simulink model "stepRecovery"  (Simulink 8.8)
settings: Solver=FixedStepDiscrete  StartTime=0.0  StopTime="CONFIG.SIMULATION_TIME "  FixedStep=CONFIG.Ts  RelTol=1e-3
InitFcn:
  | cd(fileparts(which(bdroot)));
  | initStepRecovery;
undefined symbols (not defined in the file or in its folder): bVectorConstraints, bVectorConstraintsMPC, CONFIG, ConstraintsMatrix, ConstraintsMatrixMPC, DiscIntNeverNeededParam, gain, mpc_init, reg, ROBOT_DOF, ROBOT_DOF_FOR_SIMULINK, sat, sm, WBT_robotName
libraries: WBToolboxLibrary x112, simulink x13, simulink_extras x4
(part 1 of 4)
settings Model: SuppressorTable=22 serialization::archive 11 0 3 0 0 0 11 0  Creator=daniele  LastModifiedBy=sdafarra
settings DataIOCC: SignalLoggingSaveFormat=Dataset
settings OptimizationCC: ExpressionDepthLimit=2147483647
settings DebuggingCC: SignalInfNanChecking=warning  UnderspecifiedInitializationDetection=Simplified  MergeDetectMultiDrivingBlocksExec=error  SolverPrmCheckMsg=warning  MultiTaskCondExecSysMsg=warning  SingleTaskRateTransMsg=warning  CheckMatrixSingularityMsg=warning  AllowSymbolicDim=off
settings SFSimCC: SimParseCustomCode=off

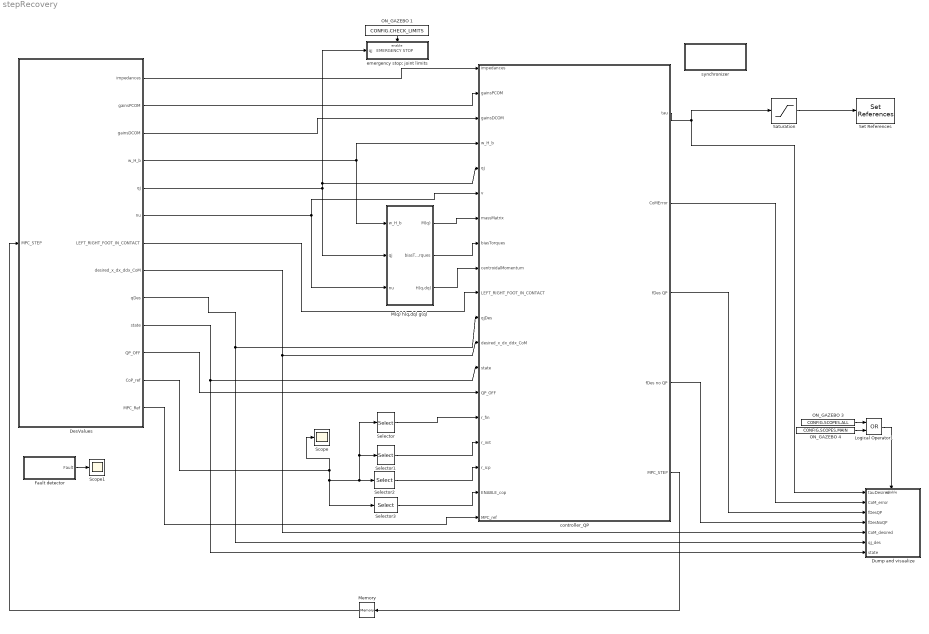
== system stepRecovery ==
  DesValues : Subsystem  Priority=-10
  Dump and visualize : Subsystem
  Fault detector : Subsystem
  Logical Operator1 : Logic  Operator=OR  AllPortsSameDT=off  OutDataTypeStr=boolean
  M(q) h(q,dq) g(q) : Subsystem
  Memory : Memory
  ON_GAZEBO 1 : Constant  Value=CONFIG.CHECK_LIMITS
  ON_GAZEBO 3 : Constant  Value=CONFIG.SCOPES.ALL
  ON_GAZEBO 4 : Constant  Value=CONFIG.SCOPES.MAIN
  Saturation : Saturate  UpperLimit=sat.torque  LowerLimit=-sat.torque
  Scope : Scope
  Scope1 : Scope
  Selector : Selector  InputPortWidth=10  IndexOptions=Index vector (dialog)  Indices=[1:3]  OutputSizes=1
  Selector1 : Selector  InputPortWidth=10  IndexOptions=Index vector (dialog)  Indices=[4:6]  OutputSizes=1
  Selector2 : Selector  InputPortWidth=10  IndexOptions=Index vector (dialog)  Indices=[7:9]  OutputSizes=1
  Selector3 : Selector  InputPortWidth=10  IndexOptions=Index vector (dialog)  Indices=[10]  OutputSizes=1
  Set References : WBToolboxLibrary/wholeBodyActuators/Set References  controlType=Torque  fullOrSubControl=Full  controlledJoints=''  robotName=WBT_robotName  localName=WBT_modelName  wbiFile=WBT_wbiFilename  wbiList=WBT_wbiList
  controller_QP : Subsystem
  emergency stop: joint limits : Subsystem
  synchronizer : Subsystem
      mask Display: disp('SYNCHRONIZER')
  wires:
  M(q) h(q,dq) g(q)/1(M(q)) -> controller_QP/7(massMatrix)
  DesValues/5(qj) -> M(q) h(q,dq) g(q)/2(qj), controller_QP/5(qj), emergency stop: joint limits/1(qj   EMERGENCY STOP)
  M(q) h(q,dq) g(q)/2(biasTorques) -> controller_QP/8(biasTorques)
  M(q) h(q,dq) g(q)/3(H(q,dq)) -> controller_QP/9(centroidalMomentum)
  controller_QP/1("tau ") -> Saturation/1, Dump and visualize/1(tauDesired)
  controller_QP/2(CoMError) -> Dump and visualize/2(CoM_error)
  DesValues/9(qDes) -> Dump and visualize/6(qj_des), controller_QP/11(qjDes)
  DesValues/7(LEFT_RIGHT_FOOT_IN_CONTACT) -> controller_QP/10(LEFT_RIGHT_FOOT_IN_CONTACT)
  DesValues/8(desired_x_dx_ddx_CoM) -> Dump and visualize/5(CoM_desired), controller_QP/12(desired_x_dx_ddx_CoM)
  DesValues/1(impedances) -> controller_QP/1(impedances)
  DesValues/4(w_H_b) -> M(q) h(q,dq) g(q)/1(w_H_b), controller_QP/4(w_H_b)
  DesValues/6(nu) -> M(q) h(q,dq) g(q)/3(nu), controller_QP/6(v)
  Logical Operator1/1 -> Dump and visualize/Enable
  DesValues/10(state) -> Dump and visualize/7(state), controller_QP/13("state ")
  controller_QP/4(fDes no QP) -> Dump and visualize/4(fDesNoQP)
  controller_QP/3(fDes QP) -> Dump and visualize/3(fDesQP)
  ON_GAZEBO 1/1 -> emergency stop: joint limits/Enable
  ON_GAZEBO 3/1 -> Logical Operator1/1
  ON_GAZEBO 4/1 -> Logical Operator1/2
  DesValues/2(gainsPCOM) -> controller_QP/2(gainsPCOM)
  DesValues/3(gainsDCOM) -> controller_QP/3(gainsDCOM)
  DesValues/11("QP_OFF ") -> controller_QP/14(QP_OFF)
  Saturation/1 -> Set References/1
  Selector2/1 -> controller_QP/17(r_icp)
  Selector1/1 -> controller_QP/16(r_init)
  Selector/1 -> controller_QP/15(r_fin)
  Selector3/1 -> controller_QP/18(ENABLE_cop)
  DesValues/12(CoP_ref) -> Selector1/1, Selector/1, Selector2/1, Selector3/1, Scope/1
  DesValues/13(MPC_Ref) -> controller_QP/19(MPC_ref)
  Fault detector/1("Fault ") -> Scope1/1
  controller_QP/5(MPC_STEP) -> Memory/1
  Memory/1 -> DesValues/1(MPC_STEP)

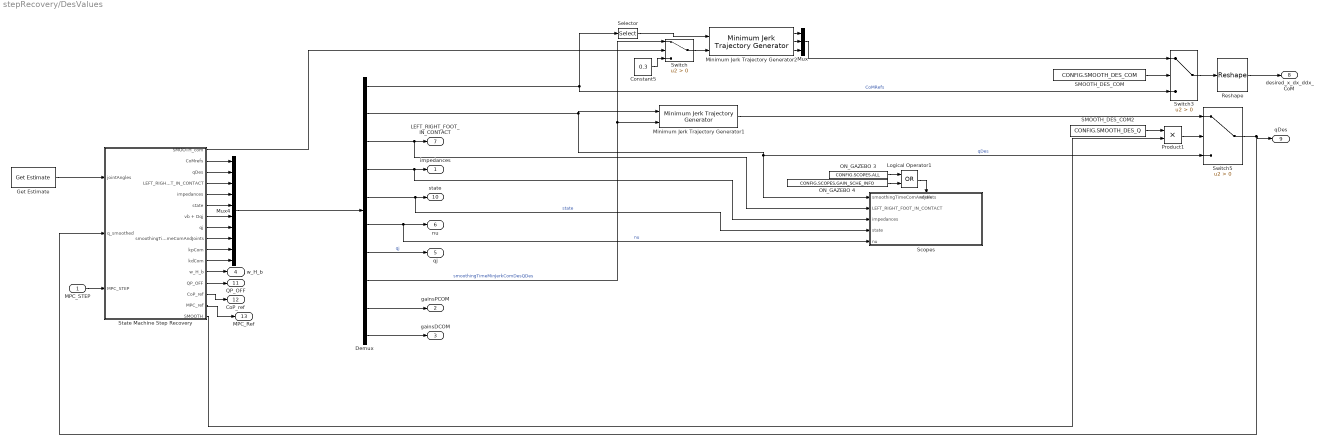
== system stepRecovery/DesValues ==
  MPC_STEP : Inport
  Constant5 : Constant  Value=0.3
  Demux : Demux  Outputs=[9,ROBOT_DOF,2,ROBOT_DOF,1,ROBOT_DOF+6,ROBOT_DOF,1,3,3]
  Get Estimate : WBToolboxLibrary/wholeBodyStates/Get Estimate  estimateType=Joints Position  robotName=WBT_robotName  localName=WBT_modelName  wbiFile=WBT_wbiFilename  wbiList=WBT_wbiList
  Logical Operator1 : Logic  Operator=OR  AllPortsSameDT=off  OutDataTypeStr=boolean
  Minimum Jerk Trajectory Generator1 : WBToolboxLibrary/Utilities/Minimum Jerk Trajectory Generator  externalSettlingTime=on  settlingTime=1  sampleTime=CONFIG.Ts  resetOnSettlingTime=off  firstDerivatives=off  secondDerivatives=off  explicitInitialValue=off
  Minimum Jerk Trajectory Generator2 : WBToolboxLibrary/Utilities/Minimum Jerk Trajectory Generator  externalSettlingTime=on  settlingTime=references.com.smoothingTime  sampleTime=CONFIG.Ts  resetOnSettlingTime=off  firstDerivatives=on  secondDerivatives=on  explicitInitialValue=off
  Mux : Mux  Inputs=3
  Mux4 : Mux  Inputs=10
  ON_GAZEBO 3 : Constant  Value=CONFIG.SCOPES.ALL
  ON_GAZEBO 4 : Constant  Value=CONFIG.SCOPES.GAIN_SCHE_INFO
  Product1 : Product
  Reshape : Reshape  OutputDimensionality=Customize  OutputDimensions=[3,3]
  SMOOTH_DES_COM : Constant  Value=CONFIG.SMOOTH_DES_COM
  SMOOTH_DES_COM2 : Constant  Value=CONFIG.SMOOTH_DES_Q
  "Scopes  " : Subsystem
  Selector : Selector  InputPortWidth=9  IndexOptions=Index vector (dialog)  Indices=[1 2 3]  OutputSizes=1
  State Machine Step Recovery : Subsystem  Priority=-100
  Switch : Switch  Criteria=u2 > Threshold
  Switch3 : Switch  Criteria=u2 > Threshold
  Switch5 : Switch  Criteria=u2 > Threshold
  impedances : Outport
  gainsPCOM : Outport  Port=2
  gainsDCOM : Outport  Port=3
  w_H_b : Outport  Port=4
  qj : Outport  Port=5
  nu : Outport  Port=6
  LEFT_RIGHT_FOOT_IN_CONTACT : Outport  Port=7
  desired_x_dx_ddx_CoM : Outport  Port=8
  qDes : Outport  Port=9
  state : Outport  Port=10
  "QP_OFF " : Outport  Port=11
  CoP_ref : Outport  Port=12
  MPC_Ref : Outport  Port=13
  wires:
  Reshape/1 -> desired_x_dx_ddx_CoM/1
  Minimum Jerk Trajectory Generator2/1 -> Mux/1
  Minimum Jerk Trajectory Generator2/2 -> Mux/2
  Minimum Jerk Trajectory Generator2/3 -> Mux/3
  Switch3/1 -> Reshape/1
  Switch5/1 -> State Machine Step Recovery/2("q_smoothed "), qDes/1
  Demux/7 -> qj/1  "qj"
  State Machine Step Recovery/12(w_H_b) -> w_H_b/1
  Demux/5 -> "Scopes  "/4(state), state/1  "state"
  Demux/8 -> Switch/1, Minimum Jerk Trajectory Generator1/2  "smoothingTimeMinJerkComDesQDes"
  Logical Operator1/1 -> "Scopes  "/Enable
  Demux/1 -> Selector/1, Switch3/3  "CoMRefs"
  Mux/1 -> Switch3/1
  Selector/1 -> Minimum Jerk Trajectory Generator2/1
  Demux/2 -> Minimum Jerk Trajectory Generator1/1, "Scopes  "/1(smoothingTimeComAndJoints), Switch5/3  "qDes"
  Minimum Jerk Trajectory Generator1/1 -> Switch5/1
  ON_GAZEBO 3/1 -> Logical Operator1/1
  ON_GAZEBO 4/1 -> Logical Operator1/2
  Demux/6 -> nu/1, "Scopes  "/5(nu)  "nu"
  Mux4/1 -> Demux/1
  Demux/4 -> "Scopes  "/3(impedances), impedances/1
  Demux/3 -> "Scopes  "/2(LEFT_RIGHT_FOOT_IN_CONTACT), LEFT_RIGHT_FOOT_IN_CONTACT/1
  Demux/9 -> gainsPCOM/1
  Demux/10 -> gainsDCOM/1
  State Machine Step Recovery/4(LEFT_RIGHT_FOOT_IN_CONTACT) -> Mux4/3
  State Machine Step Recovery/3(qDes) -> Mux4/2
  State Machine Step Recovery/2(CoMrefs) -> Mux4/1
  State Machine Step Recovery/5(impedances) -> Mux4/4
  State Machine Step Recovery/6(state) -> Mux4/5
  State Machine Step Recovery/7(vb + Dqj) -> Mux4/6
  State Machine Step Recovery/8(qj) -> Mux4/7
  State Machine Step Recovery/9(smoothingTimeComAndJoints) -> Mux4/8
  Get Estimate/1 -> State Machine Step Recovery/1(jointAngles)
  State Machine Step Recovery/10(kpCom) -> Mux4/9
  State Machine Step Recovery/11(kdCom) -> Mux4/10
  State Machine Step Recovery/13(QP_OFF) -> "QP_OFF "/1
  SMOOTH_DES_COM/1 -> Switch3/2
  SMOOTH_DES_COM2/1 -> Product1/1
  Product1/1 -> Switch5/2
  State Machine Step Recovery/16(SMOOTH) -> Product1/2
  State Machine Step Recovery/1(SMOOTH_com) -> Switch/2
  Switch/1 -> Minimum Jerk Trajectory Generator2/2
  Constant5/1 -> Switch/3
  State Machine Step Recovery/14(CoP_ref) -> CoP_ref/1
  State Machine Step Recovery/15(MPC_ref) -> MPC_Ref/1
  MPC_STEP/1 -> State Machine Step Recovery/3(MPC_STEP)

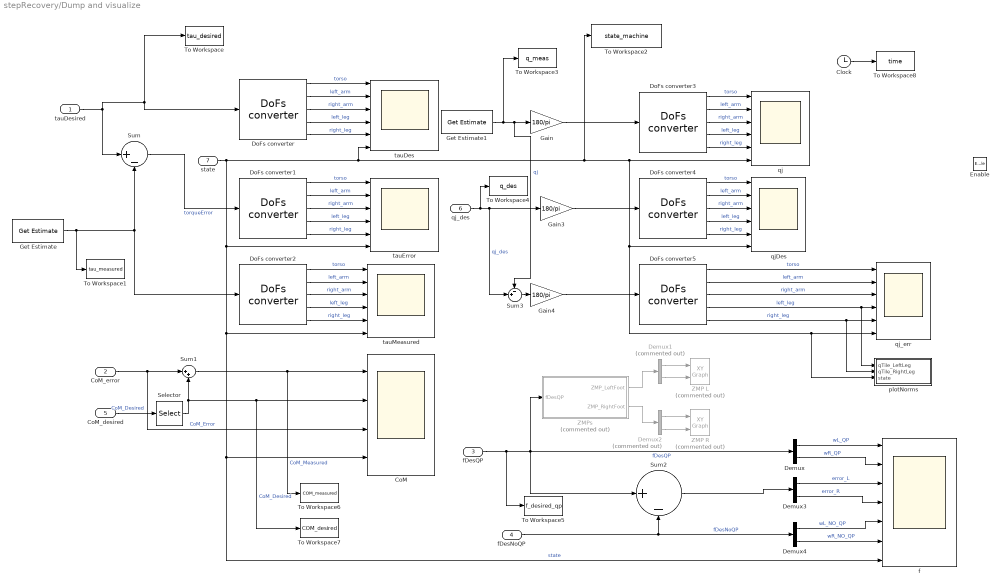
== system stepRecovery/Dump and visualize ==
  tauDesired : Inport
  CoM_error : Inport  Port=2
  fDesQP : Inport  Port=3
  fDesNoQP : Inport  Port=4
  CoM_desired : Inport  Port=5
  qj_des : Inport  Port=6
  state : Inport  Port=7
  Enable : EnablePort
  Clock : Clock
  CoM : Scope  NumInputPorts=4
  Demux : Demux  Outputs=2
  Demux1 : Demux  Commented=on  Outputs=2
  Demux2 : Demux  Commented=on  Outputs=2
  Demux3 : Demux  Outputs=2
  Demux4 : Demux  Outputs=2
  DoFs converter{,1..5} (6 alike) : WBToolboxLibrary/Utilities/DoFs converter  yarp2WBIOption=From WBI to YARP  robotName=WBT_robotName  localName=WBT_modelName  wbiFile=WBT_wbiFilename  wbiList=WBT_wbiList
  Gain : Gain  Gain=180/pi
  Gain3 : Gain  Gain=180/pi
  Gain4 : Gain  Gain=180/pi
  Get Estimate : WBToolboxLibrary/wholeBodyStates/Get Estimate  estimateType=Joints Torque  robotName=WBT_robotName  localName=WBT_modelName  wbiFile=WBT_wbiFilename  wbiList=WBT_wbiList
  Get Estimate1 : WBToolboxLibrary/wholeBodyStates/Get Estimate  estimateType=Joints Position  robotName=WBT_robotName  localName=WBT_modelName  wbiFile=WBT_wbiFilename  wbiList=WBT_wbiList
  Selector : Selector  NumberOfDimensions=2  IndexOptions=Index vector (dialog),Index vector (dialog)  Indices=[1:3],1  OutputSizes=1,1
  Sum : Sum  Inputs=|+-
  Sum1 : Sum  Inputs=|++
  Sum2 : Sum  Inputs=|+-
  Sum3 : Sum  Inputs=-+|
  To Workspace : ToWorkspace  VariableName=tau_desired  SampleTime=-1
      settings: Save2DSignal=2-D array (concatenate along first dimension)
  To Workspace1 : ToWorkspace  VariableName=tau_measured  SampleTime=-1
      settings: Save2DSignal=2-D array (concatenate along first dimension)
  To Workspace2 : ToWorkspace  VariableName=state_machine  SampleTime=-1
  To Workspace3 : ToWorkspace  VariableName=q_meas  SampleTime=-1
  To Workspace4 : ToWorkspace  VariableName=q_des  SampleTime=-1
  To Workspace5 : ToWorkspace  VariableName=f_desired_qp  SampleTime=-1
      settings: Save2DSignal=2-D array (concatenate along first dimension)
  To Workspace6 : ToWorkspace  VariableName=COM_measured  SampleTime=-1
  To Workspace7 : ToWorkspace  VariableName=COM_desired  SampleTime=-1
  To Workspace8 : ToWorkspace  VariableName=time  SampleTime=-1
  ZMP L : simulink/Sinks/XY Graph  Commented=on  xmin=gain.footSize(1,1)  xmax=gain.footSize(1,2)  ymin=gain.footSize(2,1)  ymax=gain.footSize(2,2)  st=-1
  ZMP R : simulink/Sinks/XY Graph  Commented=on  xmin=gain.footSize(1,1)  xmax=gain.footSize(1,2)  ymin=gain.footSize(2,1)  ymax=gain.footSize(2,2)  st=-1
  ZMPs : Subsystem  Commented=on
  f : Scope  NumInputPorts=7
  plotNorms : Subsystem
  qj : Scope  NumInputPorts=6
  qjDes : Scope  NumInputPorts=6
  qj_err : Scope  NumInputPorts=6
  tauDes : Scope  NumInputPorts=6
  tauError : Scope  NumInputPorts=6
  tauMeasured : Scope  NumInputPorts=6
  wires:
  CoM_error/1 -> Sum1/1, CoM/3  "CoM_Error"
  CoM_desired/1 -> Selector/1  "CoM_Desired"
  Sum1/1 -> To Workspace6/1, CoM/1  "CoM_Measured"
  Get Estimate1/1 -> To Workspace3/1, Sum3/1, Gain/1  "qj"
  Gain/1 -> DoFs converter3/1
  DoFs converter3/5 -> qj/5  "right_leg"
  DoFs converter3/1 -> qj/1  "torso"
  DoFs converter3/2 -> qj/2  "left_arm"
  DoFs converter3/4 -> qj/4  "left_leg"
  DoFs converter3/3 -> qj/3  "right_arm"
  fDesQP/1 -> To Workspace5/1, Demux/1, ZMPs/1(fDesQP), Sum2/1  "fDesQP"
  ZMPs/1(ZMP_LeftFoot) -> Demux1/1
  ZMPs/2(ZMP_RightFoot) -> Demux2/1
  Demux1/1 -> ZMP L/1
  Demux1/2 -> ZMP L/2
  Demux2/1 -> ZMP R/1
  Demux2/2 -> ZMP R/2
  Sum2/1 -> Demux3/1
  fDesNoQP/1 -> Demux4/1, Sum2/2  "fDesNoQP"
  tauDesired/1 -> DoFs converter/1, To Workspace/1, Sum/1
  Get Estimate/1 -> To Workspace1/1, DoFs converter2/1, Sum/2
  DoFs converter/5 -> tauDes/5  "right_leg"
  DoFs converter/1 -> tauDes/1  "torso"
  DoFs converter/2 -> tauDes/2  "left_arm"
  DoFs converter/4 -> tauDes/4  "left_leg"
  DoFs converter/3 -> tauDes/3  "right_arm"
  DoFs converter1/5 -> tauError/5  "right_leg"
  DoFs converter1/1 -> tauError/1  "torso"
  DoFs converter1/2 -> tauError/2  "left_arm"
  DoFs converter1/4 -> tauError/4  "left_leg"
  DoFs converter1/3 -> tauError/3  "right_arm"
  Sum/1 -> DoFs converter1/1  "torqueError"
  DoFs converter2/5 -> tauMeasured/5  "right_leg"
  DoFs converter2/1 -> tauMeasured/1  "torso"
  DoFs converter2/2 -> tauMeasured/2  "left_arm"
  DoFs converter2/4 -> tauMeasured/4  "left_leg"
  DoFs converter2/3 -> tauMeasured/3  "right_arm"
  qj_des/1 -> To Workspace4/1, Sum3/2, Gain3/1  "qj_des"
  Gain3/1 -> DoFs converter4/1
  DoFs converter4/5 -> qjDes/5  "right_leg"
  DoFs converter4/1 -> qjDes/1  "torso"
  DoFs converter4/2 -> qjDes/2  "left_arm"
  DoFs converter4/4 -> qjDes/4  "left_leg"
  DoFs converter4/3 -> qjDes/3  "right_arm"
  Gain4/1 -> DoFs converter5/1
  DoFs converter5/5 -> plotNorms/2(qTile_RightLeg), qj_err/5  "right_leg"
  DoFs converter5/1 -> qj_err/1  "torso"
  DoFs converter5/2 -> qj_err/2  "left_arm"
  DoFs converter5/4 -> plotNorms/1(qTile_LeftLeg), qj_err/4  "left_leg"
  DoFs converter5/3 -> qj_err/3  "right_arm"
  Sum3/1 -> Gain4/1
  Selector/1 -> Sum1/2, To Workspace7/1, CoM/2  "CoM_Desired"
  state/1 -> tauDes/6, To Workspace2/1, plotNorms/3(state), qj_err/6, qjDes/6, qj/6, f/7, CoM/4, tauMeasured/6, tauError/6  "state"
  Demux/1 -> f/1  "wL_QP"
  Demux/2 -> f/2  "wR_QP"
  Demux3/1 -> f/3  "error_L"
  Demux3/2 -> f/4  "error_R"
  Demux4/1 -> f/5  "wL_NO_QP"
  Demux4/2 -> f/6  "wR_NO_QP"
  Clock/1 -> To Workspace8/1

== system stepRecovery/Fault detector ==
  Abs : Abs
  Compare To Constant : simulink/Logic and Bit Operations/Compare To Constant  relop=>=  const=0.1  OutDataTypeStr=boolean
  Compare To Constant1 : simulink/Logic and Bit Operations/Compare To Constant  relop=<  const=1  OutDataTypeStr=boolean
  Data Type Conversion : DataTypeConversion  OutDataTypeStr=int8
  Sum of Elements : Sum  Inputs=+  OutDataTypeStr=int8
  chest_wrench : WBToolboxLibrary/Utilities/Yarp Read  portName='/controlBoardDumper/left_leg/getMotorsPwm'  signalSize=6  blocking=off  timestamp=off  autoconnect=on  errorOnConnection=off
  "Fault " : Outport
  wires:
  Abs/1 -> Compare To Constant/1
  Sum of Elements/1 -> Compare To Constant1/1
  chest_wrench/1 -> Abs/1
  Data Type Conversion/1 -> Sum of Elements/1
  Compare To Constant/1 -> Data Type Conversion/1
  Compare To Constant1/1 -> "Fault "/1

== system stepRecovery/M(q) h(q,dq) g(q) ==
  w_H_b : Inport
  qj : Inport  Port=2
  nu : Inport  Port=3
  Centroidal Momentum : WBToolboxLibrary/wholeBodyModel/Dynamics/Centroidal Momentum  robotName=WBT_robotName  localName=WBT_modelName  wbiFile=WBT_wbiFilename  wbiList=WBT_wbiList
  "CoM6D ->  CoMXYZ1" : Selector  InputPortWidth=6+ROBOT_DOF  IndexOptions=Index vector (dialog)  Indices=[7:6+ROBOT_DOF]  OutputSizes=1
  "CoM6D ->  CoMXYZ2" : Selector  InputPortWidth=6+ROBOT_DOF  IndexOptions=Index vector (dialog)  Indices=[1 2 3 4 5 6]  OutputSizes=1
  Get Bias Forces : WBToolboxLibrary/wholeBodyModel/Dynamics/Get Bias Forces  robotName=WBT_robotName  localName=WBT_modelName  wbiFile=WBT_wbiFilename  wbiList=WBT_wbiList  explicitGravity=off
  Mass Matrix : WBToolboxLibrary/wholeBodyModel/Dynamics/Mass Matrix  robotName=WBT_robotName  localName=WBT_modelName  wbiFile=WBT_wbiFilename  wbiList=WBT_wbiList
  M(q) : Outport
  biasTorques : Outport  Port=2
  H(q,dq) : Outport  Port=3
  wires:
  Mass Matrix/1 -> M(q)/1
  Centroidal Momentum/1 -> H(q,dq)/1
  Get Bias Forces/1 -> biasTorques/1
  w_H_b/1 -> Centroidal Momentum/1, Get Bias Forces/1, Mass Matrix/1
  qj/1 -> Centroidal Momentum/2, Get Bias Forces/2, Mass Matrix/2
  "CoM6D ->  CoMXYZ2"/1 -> Centroidal Momentum/3, Get Bias Forces/3
  "CoM6D ->  CoMXYZ1"/1 -> Get Bias Forces/4, Centroidal Momentum/4
  nu/1 -> "CoM6D ->  CoMXYZ1"/1, "CoM6D ->  CoMXYZ2"/1

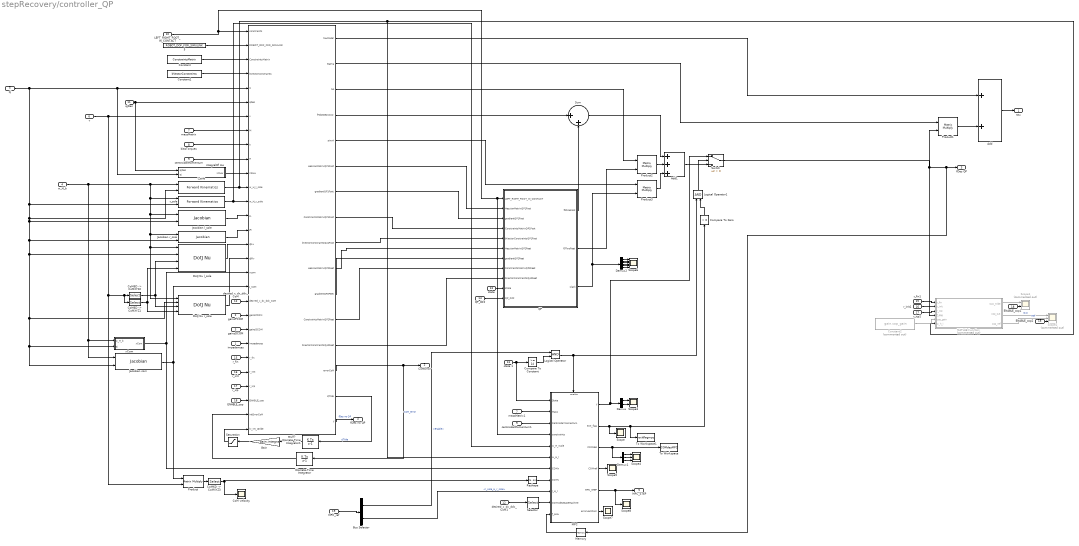
== system stepRecovery/controller_QP ==
  impedances : Inport
  gainsPCOM : Inport  Port=2
  gainsDCOM : Inport  Port=3
  w_H_b : Inport  Port=4
  qj : Inport  Port=5
  v : Inport  Port=6
  massMatrix : Inport  Port=7
  biasTorques : Inport  Port=8
  centroidalMomentum : Inport  Port=9
  LEFT_RIGHT_FOOT_IN_CONTACT : Inport  Port=10
  qjDes : Inport  Port=11
  desired_x_dx_ddx_CoM : Inport  Port=12
  "state " : Inport  Port=13
  QP_OFF : Inport  Port=14
  r_fin : Inport  Port=15
  r_init : Inport  Port=16
  r_icp : Inport  Port=17
  ENABLE_cop : Inport  Port=18
  MPC_ref : Inport  Port=19
  "    5" : Constant  Value=ROBOT_DOF_FOR_SIMULINK
  Add : Sum
  Add1 : Sum  Inputs=+++
  Bus Selector : BusSelector  OutputSignals=Enable,l_sole_H_r_sole
  CoM velocity : Scope
  "CoM6D ->  CoMXYZ1" : Selector  InputPortWidth=6+ROBOT_DOF  IndexOptions=Index vector (dialog)  Indices=[7:6+ROBOT_DOF]  OutputSizes=1
  "CoM6D ->  CoMXYZ2" : Selector  InputPortWidth=6+ROBOT_DOF  IndexOptions=Index vector (dialog)  Indices=[1 2 3 4 5 6]  OutputSizes=1
  "CoM6D ->  CoMXYZ3" : Selector  InputPortWidth=6  IndexOptions=Index vector (dialog)  Indices=[1 2 3]  OutputSizes=1
  Compare To Constant : simulink/Logic and Bit Operations/Compare To Constant  relop=>=  const=14  OutDataTypeStr=boolean
  Compare To Zero : simulink/Logic and Bit Operations/Compare To Zero  relop=>  OutDataTypeStr=boolean
  Constant : Constant  Value=ConstraintsMatrix
  Constant1 : Constant  Value=bVectorConstraints
  Constant2 : Constant  Commented=on  Value=gain.cop_gain
  Demux : Demux  Outputs=2
  Demux1 : Demux  Outputs=3
  Demux2 : Demux  Outputs=6
  Discrete-Time Integrator : DiscreteIntegrator  InitialCondition=[0 0 0]  SampleTime=CONFIG.Ts  ICPrevOutput=DiscIntNeverNeededParam  ICPrevScaledInput=DiscIntNeverNeededParam
  Discrete-Time Integrator1 : DiscreteIntegrator  InitialCondition=zeros(ROBOT_DOF,1)  SampleTime=CONFIG.Ts  ICPrevOutput=DiscIntNeverNeededParam  ICPrevScaledInput=DiscIntNeverNeededParam
  "DotJ Nu l_sole " : WBToolboxLibrary/wholeBodyModel/Jacobians/DotJ Nu  frameName='l_sole'  robotName=WBT_robotName  localName=WBT_modelName  wbiFile=WBT_wbiFilename  wbiList=WBT_wbiList
  "DotJ Nu r_sole " : WBToolboxLibrary/wholeBodyModel/Jacobians/DotJ Nu  frameName='r_sole'  robotName=WBT_robotName  localName=WBT_modelName  wbiFile=WBT_wbiFilename  wbiList=WBT_wbiList
  ENABLE_cop1 : InportShadow  Port=18
  ENABLE_cop2 : InportShadow  Port=18
  Gain : Gain  Gain=gain.integral
  Jacobian com : WBToolboxLibrary/wholeBodyModel/Jacobians/Jacobian  frameName='com'  robotName=WBT_robotName  localName=WBT_modelName  wbiFile=WBT_wbiFilename  wbiList=WBT_wbiList
  Jacobian l_sole : WBToolboxLibrary/wholeBodyModel/Jacobians/Jacobian  frameName='l_sole'  robotName=WBT_robotName  localName=WBT_modelName  wbiFile=WBT_wbiFilename  wbiList=WBT_wbiList
  Jacobian r_sole : WBToolboxLibrary/wholeBodyModel/Jacobians/Jacobian  frameName='r_sole'  robotName=WBT_robotName  localName=WBT_modelName  wbiFile=WBT_wbiFilename  wbiList=WBT_wbiList
  Logical Operator : Logic  AllPortsSameDT=off  OutDataTypeStr=boolean
  Logical Operator1 : Logic  AllPortsSameDT=off  OutDataTypeStr=boolean
  MATLAB Function : MATLAB Function  Commented=on  TreatAsAtomicUnit=on
  "MPC " : Subsystem
  Memory : Memory
  Product{,1..3} (4 alike) : Product  Multiplication=Matrix(*)
  QP : Subsystem
  Reshape : Reshape  OutputDimensionality=Column vector (2-D)
  Saturation : Saturate  UpperLimit=sat.integral  LowerLimit=-sat.integral
  Scope{,5,7..8} (4 alike) : Scope
  Scope1 : Scope  Commented=on  NumInputPorts=2
  Scope2 : Scope  Commented=on  NumInputPorts=3
  Scope3 : Scope  NumInputPorts=2
  Scope4 : Scope  NumInputPorts=3
  Scope6 : Scope  NumInputPorts=6
  Selector : Selector  NumberOfDimensions=2  InputPortWidth=3  IndexOptions=Index vector (dialog),Index vector (dialog)  Indices=[1:3],[1:2]  OutputSizes=1,1
  Sum : Sum  Inputs=|++
  "Switch " : Switch  Criteria=u2 > Threshold
  To Workspace : ToWorkspace  VariableName=COMdesMPC  SampleTime=-1
  To Workspace1 : ToWorkspace  VariableName=exitflagmpc  SampleTime=-1
  centroidalMomentum1 : InportShadow  Port=9
  desired_x_dx_ddx_CoM1 : InportShadow  Port=12
  integralOf Hw : Subsystem
  l_sole : WBToolboxLibrary/wholeBodyModel/Kinematics/Forward Kinematics  frameName='l_sole'  robotName=WBT_robotName  localName=WBT_modelName  wbiFile=WBT_wbiFilename  wbiList=WBT_wbiList
  massMatrix1 : InportShadow  Port=7
  r_fin1 : InportShadow  Port=15
  r_icp1 : InportShadow  Port=17
  r_init1 : InportShadow  Port=16
  r_sole : WBToolboxLibrary/wholeBodyModel/Kinematics/Forward Kinematics  frameName='r_sole'  robotName=WBT_robotName  localName=WBT_modelName  wbiFile=WBT_wbiFilename  wbiList=WBT_wbiList
  state 1 : InportShadow  Port=13
  "tau(f) " : MATLAB Function  TreatAsAtomicUnit=on
  xCom : Subsystem
  "tau " : Outport
  CoMError : Outport  Port=2
  fDes QP : Outport  Port=3
  fDes no QP : Outport  Port=4
  MPC_STEP : Outport  Port=5
  wires:
  LEFT_RIGHT_FOOT_IN_CONTACT/1 -> "MPC "/4("constraints "), QP/1(LEFT_RIGHT_FOOT_IN_CONTACT), "tau(f) "/1(constraints)
  Discrete-Time Integrator/1 -> "tau(f) "/28(intErrorCoM)
  "tau(f) "/14(errorCoM) -> CoMError/1, Discrete-Time Integrator/1  "CoM_Error"
  Discrete-Time Integrator1/1 -> Gain/1
  "tau(f) "/15(qTilde) -> Discrete-Time Integrator1/1  "qTilde"
  Gain/1 -> Saturation/1
  Saturation/1 -> "tau(f) "/29(ki_int_qtilde)
  qj/1 -> xCom/2(qj), Jacobian com/2, "DotJ Nu r_sole "/2, "DotJ Nu l_sole "/2, Jacobian r_sole/2, Jacobian l_sole/2, l_sole/2, r_sole/2, integralOf Hw/2(qj), "tau(f) "/5(q)
  qjDes/1 -> integralOf Hw/1(qjDes), "tau(f) "/6(qDes)
  massMatrix/1 -> "tau(f) "/8(M)
  biasTorques/1 -> "tau(f) "/9(h)
  desired_x_dx_ddx_CoM/1 -> "tau(f) "/20(desired_x_dx_ddx_CoM)
  impedances/1 -> "tau(f) "/23(impedances)
  centroidalMomentum/1 -> "tau(f) "/10(H)
  r_sole/1 -> "MPC "/5(w_H_rsole), "tau(f) "/13(w_H_r_sole)
  l_sole/1 -> "MPC "/6(w_H_l), MATLAB Function/6(w_h_l), "tau(f) "/12(w_H_l_sole)
  Jacobian l_sole/1 -> "tau(f) "/14(JL)
  Jacobian r_sole/1 -> "tau(f) "/15(JR)
  Jacobian com/1 -> "tau(f) "/19(J_CoM), Product/1
  "tau(f) "/6(HessianMatrixQP1Foot) -> QP/2(HessianMatrixQP1Foot)
  "tau(f) "/7(gradientQP1Foot) -> QP/3(gradientQP1Foot)
  "tau(f) "/10(HessianMatrixQP2Feet) -> QP/6(HessianMatrixQP2Feet)
  "tau(f) "/11(gradientQP2Feet) -> QP/7(gradientQP2Feet)
  "tau(f) "/12(ConstraintsMatrixQP2Feet) -> QP/8(ConstraintsMatrixQP2Feet)
  "tau(f) "/13(bVectorConstraintsQp2Feet) -> QP/9(bVectorConstraintsQp2Feet)
  "tau(f) "/4(fHdotDesC1C2) -> Sum/1
  QP/1(f0OneFoot) -> Sum/2
  Product1/1 -> Add/2
  "tau(f) "/1(tauModel) -> Add/1
  Add/1 -> "tau "/1
  "Switch "/1 -> MATLAB Function/4(f_qpg), Product1/2, Memory/1, fDes QP/1
  "    5"/1 -> "tau(f) "/2(ROBOT_DOF_FOR_SIMULINK)
  Constant/1 -> "tau(f) "/3(ConstraintsMatrix)
  Constant1/1 -> "tau(f) "/4(bVectorConstraints)
  "tau(f) "/8(ConstraintsMatrixQP1Foot) -> QP/4(ConstraintsMatrixQP1Foot)
  "tau(f) "/9(bVectorConstraintsQp1Foot) -> QP/5(bVectorConstraintsQP1Foot)
  Sum/1 -> Add1/1
  Product2/1 -> Add1/2
  "tau(f) "/3(NA) -> Product2/1
  "tau(f) "/2(Sigma) -> Product1/1
  "tau(f) "/16(f) -> fDes no QP/1  "fDes no QP"
  "DotJ Nu l_sole "/1 -> "tau(f) "/16(dJLv)
  "DotJ Nu r_sole "/1 -> "tau(f) "/17(dJRv)
  xCom/1(xCom) -> "MPC "/7("COMx "), "tau(f) "/18(xcom)
  "CoM6D ->  CoMXYZ2"/1 -> "DotJ Nu r_sole "/3, "DotJ Nu l_sole "/3
  "CoM6D ->  CoMXYZ1"/1 -> "DotJ Nu r_sole "/4, "DotJ Nu l_sole "/4
  w_H_b/1 -> xCom/1(w_H_b), Jacobian com/1, "DotJ Nu r_sole "/1, "DotJ Nu l_sole "/1, Jacobian r_sole/1, Jacobian l_sole/1, r_sole/1, l_sole/1
  QP/2(f0TwoFeet) -> Product2/2
  integralOf Hw/1(intHw) -> "tau(f) "/11(intHw)
  "state "/1 -> QP/10(state)
  v/1 -> Product/2, "CoM6D ->  CoMXYZ1"/1, "CoM6D ->  CoMXYZ2"/1, "tau(f) "/7(v)
  Product/1 -> "CoM6D ->  CoMXYZ3"/1
  gainsPCOM/1 -> "tau(f) "/21(gainsPCOM)
  gainsDCOM/1 -> "tau(f) "/22(gainsDCOM)
  QP_OFF/1 -> QP/11(QP_OFF)
  r_fin/1 -> "tau(f) "/24(r_fin)
  r_init/1 -> "tau(f) "/25(r_init)
  r_icp/1 -> "tau(f) "/26(r_icp)
  ENABLE_cop/1 -> "tau(f) "/27(ENABLE_cop)
  MATLAB Function/1(icpx_tilde) -> Scope1/1
  r_fin1/1 -> MATLAB Function/1(r_fin)
  r_init1/1 -> MATLAB Function/2(r_init)
  r_icp1/1 -> MATLAB Function/3(r_icp)
  ENABLE_cop1/1 -> Scope1/2
  Constant2/1 -> MATLAB Function/5(cop_gain)
  MATLAB Function/2(cop_out) -> Scope2/1  "Out"
  ENABLE_cop2/1 -> Scope2/3
  MATLAB Function/3(cop_ref) -> Scope2/2  "Ref"
  "CoM6D ->  CoMXYZ3"/1 -> Reshape/1, CoM velocity/1
  centroidalMomentum1/1 -> "MPC "/3(Centroidal Momentum)
  massMatrix1/1 -> "MPC "/2(Mass)
  Compare To Constant/1 -> Logical Operator/2
  state 1/1 -> "MPC "/1(State), Compare To Constant/1
  MPC_ref/1 -> Bus Selector/1
  Bus Selector/2 -> "MPC "/9(l_H_r)  "<l_sole_H_r_sole>"
  Bus Selector/1 -> Logical Operator/1  "<Enable>"
  "MPC "/3(COMdes) -> Demux1/1, To Workspace/1
  "MPC "/1(f) -> "Switch "/1, Demux/1
  Demux/2 -> Scope3/2
  Demux/1 -> Scope3/1
  Demux1/3 -> Scope4/3
  Demux1/2 -> Scope4/2
  Demux1/1 -> Scope4/1
  Reshape/1 -> "MPC "/8(COMv)
  Logical Operator1/1 -> "Switch "/2
  Compare To Zero/1 -> Logical Operator1/2
  Memory/1 -> "MPC "/11(f_prev)
  "MPC "/2("exit_flag ") -> Scope/1, To Workspace1/1, Compare To Zero/1
  "MPC "/4(COMref) -> Scope5/1
  desired_x_dx_ddx_CoM1/1 -> Selector/1
  Selector/1 -> "MPC "/10(COMxdesStateMachine)
  Logical Operator/1 -> "MPC "/Enable, Logical Operator1/1
  Product3/1 -> Add1/3
  QP/3(slack) -> Product3/2, Demux2/1
  "tau(f) "/5(pinvA) -> Product3/1
  Demux2/1 -> Scope6/1
  Demux2/2 -> Scope6/2
  Demux2/3 -> Scope6/3
  Demux2/4 -> Scope6/4
  Demux2/5 -> Scope6/5
  Demux2/6 -> Scope6/6
  Add1/1 -> "Switch "/3
  "MPC "/6(errorLastCom) -> Scope7/1
  "MPC "/5(MPC_STEP) -> Scope8/1, MPC_STEP/1

== system stepRecovery/emergency stop: joint limits ==
  qj   EMERGENCY STOP : Inport
  Enable : EnablePort
  Assertion : Assertion
  Get Limits : WBToolboxLibrary/wholeBodyStates/Get Limits  limitsType=Position  robotName=WBT_robotName  localName=WBT_modelName  wbiFile=WBT_wbiFilename  wbiList=WBT_wbiList
  MATLAB Function : MATLAB Function  TreatAsAtomicUnit=on
  index1 : Constant  Value=0.01  VectorParams1D=off
  wires:
  Get Limits/1 -> MATLAB Function/1(umin)
  Get Limits/2 -> MATLAB Function/2(umax)
  index1/1 -> MATLAB Function/4(tol)
  qj   EMERGENCY STOP/1 -> MATLAB Function/3(u)
  MATLAB Function/1(inRange) -> Assertion/1

== system stepRecovery/synchronizer ==
  GAZEBO_SYNCHRONIZER : Subsystem
  Logical Operator : Logic  Operator=NOT  AllPortsSameDT=off  OutDataTypeStr=boolean
  "ON_GAZEBO " : Constant  Value=CONFIG.ON_GAZEBO
  REAL_TIME_SYNC : Subsystem
  wires:
  Logical Operator/1 -> REAL_TIME_SYNC/Enable
  "ON_GAZEBO "/1 -> GAZEBO_SYNCHRONIZER/Enable, Logical Operator/1

== system stepRecovery/DesValues/Scopes   ==
  smoothingTimeComAndJoints : Inport
  LEFT_RIGHT_FOOT_IN_CONTACT : Inport  Port=2
  impedances : Inport  Port=3
  state : Inport  Port=4
  nu : Inport  Port=5
  Enable : EnablePort
  Demux : Demux  Outputs=2
  DoFs converter1 : WBToolboxLibrary/Utilities/DoFs converter  yarp2WBIOption=From WBI to YARP  robotName=WBT_robotName  localName=WBT_modelName  wbiFile=WBT_wbiFilename  wbiList=WBT_wbiList
  DoFs converter3 : WBToolboxLibrary/Utilities/DoFs converter  yarp2WBIOption=From WBI to YARP  robotName=WBT_robotName  localName=WBT_modelName  wbiFile=WBT_wbiFilename  wbiList=WBT_wbiList
  Gain : Gain  Gain=180/pi
  Gain1 : Gain  Gain=180/pi
  Impedances(t) : Scope  NumInputPorts=6
  Left right foot in contact : Scope
  Selector1 : Selector  InputPortWidth=6+ROBOT_DOF  IndexOptions=Index vector (dialog)  Indices=[7:6+ROBOT_DOF]  OutputSizes=1
  Selector2 : Selector  InputPortWidth=6+ROBOT_DOF  IndexOptions=Index vector (dialog)  Indices=[1:6]  OutputSizes=1
  jointsSmoothingTime : Scope  NumInputPorts=2
  linear and angular  base velocity : Scope  NumInputPorts=3
  "qjDot(t) " : Scope  NumInputPorts=6
  wires:
  state/1 -> "qjDot(t) "/6, linear and angular  base velocity/3, Impedances(t)/6, jointsSmoothingTime/2  "state"
  LEFT_RIGHT_FOOT_IN_CONTACT/1 -> Left right foot in contact/1  "Left right foot in contact"
  impedances/1 -> DoFs converter3/1
  smoothingTimeComAndJoints/1 -> jointsSmoothingTime/1  "smoothingTimeComAndJoints"
  DoFs converter3/4 -> Impedances(t)/4  "left_leg"
  DoFs converter3/5 -> Impedances(t)/5  "right_leg"
  DoFs converter3/3 -> Impedances(t)/3  "right_arm"
  DoFs converter3/1 -> Impedances(t)/1  "torso"
  DoFs converter3/2 -> Impedances(t)/2  "left_arm"
  Selector1/1 -> Gain/1
  DoFs converter1/4 -> "qjDot(t) "/4  "left_leg"
  DoFs converter1/5 -> "qjDot(t) "/5  "right_leg"
  DoFs converter1/3 -> "qjDot(t) "/3  "right_arm"
  DoFs converter1/1 -> "qjDot(t) "/1  "torso"
  DoFs converter1/2 -> "qjDot(t) "/2  "left_arm"
  nu/1 -> Selector1/1, Selector2/1
  Selector2/1 -> Demux/1
  Demux/1 -> linear and angular  base velocity/1  "vb"
  Demux/2 -> Gain1/1  "wb"
  Gain/1 -> DoFs converter1/1
  Gain1/1 -> linear and angular  base velocity/2

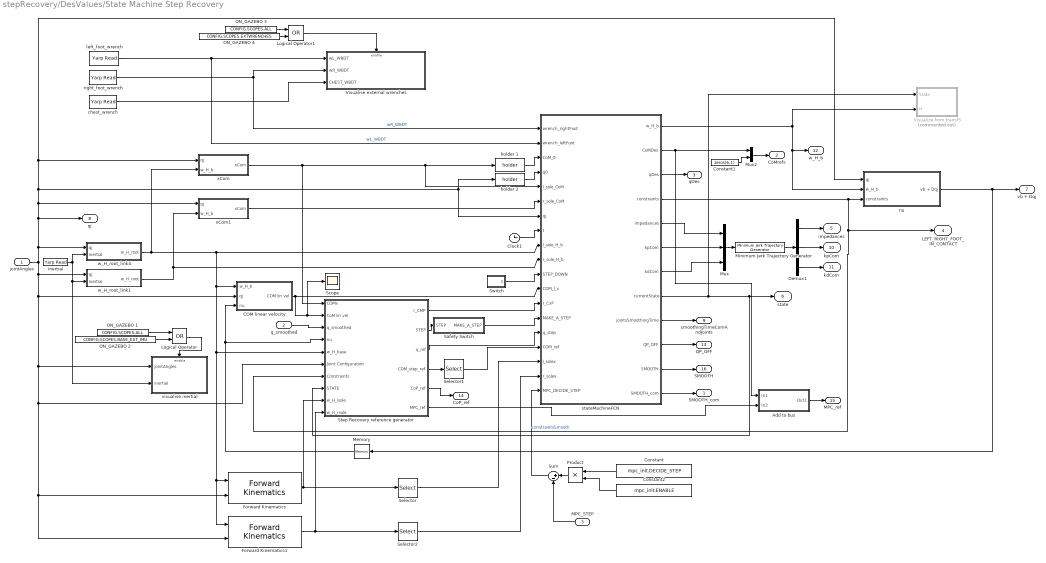
== system stepRecovery/DesValues/State Machine Step Recovery ==
  jointAngles : Inport
  "q_smoothed " : Inport  Port=2
  MPC_STEP : Inport  Port=3
  Add to bus : Subsystem
  COM linear velocity : Subsystem
  Clock1 : Clock
  Constant : Constant  Value=mpc_init.DECIDE_STEP
  Constant1 : Constant  Value=zeros(6,1)
  Constant2 : Constant  Value=mpc_init.ENABLE
  Demux1 : Demux  Outputs=[ROBOT_DOF,3,3]
  Forward Kinematics : WBToolboxLibrary/wholeBodyModel/Kinematics/Forward Kinematics  frameName='l_sole'  robotName=WBT_robotName  localName=WBT_modelName  wbiFile=WBT_wbiFilename  wbiList=WBT_wbiList
  Forward Kinematics1 : WBToolboxLibrary/wholeBodyModel/Kinematics/Forward Kinematics  frameName='r_sole'  robotName=WBT_robotName  localName=WBT_modelName  wbiFile=WBT_wbiFilename  wbiList=WBT_wbiList
  Logical Operator : Logic  Operator=OR  AllPortsSameDT=off  OutDataTypeStr=boolean
  Logical Operator1 : Logic  Operator=OR  AllPortsSameDT=off  OutDataTypeStr=boolean
  Memory : Memory
  Minimum Jerk Trajectory Generator : WBToolboxLibrary/Utilities/Minimum Jerk Trajectory Generator  externalSettlingTime=off  settlingTime=gain.SmoothingTimeGainScheduling  sampleTime=CONFIG.Ts  resetOnSettlingTime=off  firstDerivatives=off  secondDerivatives=off  explicitInitialValue=off
  Mux : Mux  Inputs=3
  Mux2 : Mux  Inputs=2
  ON_GAZEBO 1 : Constant  Value=CONFIG.SCOPES.ALL
  ON_GAZEBO 2 : Constant  Value=CONFIG.SCOPES.BASE_EST_IMU
  ON_GAZEBO 3 : Constant  Value=CONFIG.SCOPES.ALL
  ON_GAZEBO 4 : Constant  Value=CONFIG.SCOPES.EXTWRENCHES
  Product : Product
  Safety Switch : Subsystem
  Scope : Scope
  Selector : Selector  NumberOfDimensions=2  InputPortWidth=3  IndexOptions=Index vector (dialog),Index vector (dialog)  Indices=[1:3],4  OutputSizes=1,1
  Selector1 : Selector  NumberOfDimensions=2  InputPortWidth=3  IndexOptions=Index vector (dialog),Index vector (dialog)  Indices=[1:3],4  OutputSizes=1,1
  Selector2 : Selector  NumberOfDimensions=2  InputPortWidth=3  IndexOptions=Index vector (dialog),Index vector (dialog)  Indices=[1:3],4  OutputSizes=1,1
  Step Recovery reference generator : Subsystem
  Sum : Sum  Inputs=|+-
  Switch : Subsystem
  "Visualise external wrenches  " : Subsystem
  Visualize hom transf5 : Subsystem  Commented=on
  chest_wrench : WBToolboxLibrary/Utilities/Yarp Read  portName=PORTS.WBDT_CHEST  signalSize=6  blocking=off  timestamp=off  autoconnect=on  errorOnConnection=on
  holder 1 : WBToolboxLibrary/Utilities/holder 
  holder 2 : WBToolboxLibrary/Utilities/holder 
  inertial : WBToolboxLibrary/Utilities/Yarp Read  portName=PORTS.IMU  signalSize=12  blocking=off  timestamp=off  autoconnect=on  errorOnConnection=on
  left_foot_wrench : WBToolboxLibrary/Utilities/Yarp Read  portName=PORTS.WBDT_LEFTLEG_EE  signalSize=6  blocking=off  timestamp=off  autoconnect=on  errorOnConnection=on
  nu : Subsystem
  right_foot_wrench : WBToolboxLibrary/Utilities/Yarp Read  portName=PORTS.WBDT_RIGHTLEG_EE  signalSize=6  blocking=off  timestamp=off  autoconnect=on  errorOnConnection=on
  stateMachineFCN : MATLAB Function  TreatAsAtomicUnit=on
  visualise inertial : Subsystem
  w_H_root_link1 : Subsystem  mask{link_name='r_sole'}
      mask prompts: link_name "link name"
      mask help:
      | This block evaluates the homogeneous transformation between the world and the root link, i.e. ^wH_b. It assumes that the link specified by the variable 'link_name' has a constant position
      | w.r.t. an inertial frame, but it can rotate arbitrarily. This rotation is retrived from the IMU sensor.
      mask Display:
      | str = strrep(link_name, '_','\_');
      | port_label('output',1,['{}^{',str '}H_{root}'],'texmode','on')
      | clear str;
      | 
      | port_label('input',1,'q_j','texmode','on')
      | 
      | port_label('input',2,'inertial','texmode','on')
  w_H_root_link4 : Subsystem  mask{link_name='l_sole'}
      mask prompts: link_name "link name"
      mask help:
      | This block evaluates the homogeneous transformation between the world and the root link, i.e. ^wH_b. It assumes that the link specified by the variable 'link_name' has a constant position
      | w.r.t. an inertial frame, but it can rotate arbitrarily. This rotation is retrived from the IMU sensor.
      mask Display:
      | str = strrep(link_name, '_','\_');
      | port_label('output',1,['{}^{',str '}H_{root}'],'texmode','on')
      | clear str;
      | 
      | port_label('input',1,'q_j','texmode','on')
      | 
      | port_label('input',2,'inertial','texmode','on')
  xCom : Subsystem
  xCom1 : Subsystem
  SMOOTH_com : Outport
  CoMrefs : Outport  Port=2
  qDes : Outport  Port=3
  LEFT_RIGHT_FOOT_IN_CONTACT : Outport  Port=4
  impedances : Outport  Port=5
  state : Outport  Port=6
  vb + Dqj : Outport  Port=7
  qj : Outport  Port=8
  smoothingTimeComAndJoints : Outport  Port=9
  kpCom : Outport  Port=10
  kdCom : Outport  Port=11
  w_H_b : Outport  Port=12
  QP_OFF : Outport  Port=13
  CoP_ref : Outport  Port=14
  MPC_ref : Outport  Port=15
  SMOOTH : Outport  Port=16
  wires:
  Demux1/2 -> kpCom/1
  Demux1/1 -> impedances/1
  Minimum Jerk Trajectory Generator/1 -> Demux1/1
  Mux/1 -> Minimum Jerk Trajectory Generator/1
  stateMachineFCN/5(impedances) -> Mux/1
  stateMachineFCN/7(kdCom) -> Mux/3
  Demux1/3 -> kdCom/1
  stateMachineFCN/6(kpCom) -> Mux/2
  ON_GAZEBO 4/1 -> Logical Operator1/2
  ON_GAZEBO 3/1 -> Logical Operator1/1
  Logical Operator/1 -> visualise inertial/Enable
  ON_GAZEBO 2/1 -> Logical Operator/2
  ON_GAZEBO 1/1 -> Logical Operator/1
  Logical Operator1/1 -> "Visualise external wrenches  "/Enable
  stateMachineFCN/9(jointsSmoothingTime) -> smoothingTimeComAndJoints/1
  inertial/1 -> visualise inertial/2(inertial), w_H_root_link1/2(inertial), w_H_root_link4/2(inertial)
  jointAngles/1 -> qj/1, xCom1/1(qj), holder 2/1, stateMachineFCN/7(qj), xCom/1(qj), nu/1(qj), w_H_root_link4/1(qj), Step Recovery reference generator/6(Joint Configuration), Forward Kinematics/2, Forward Kinematics1/2, visualise inertial/1(jointAngles), COM linear velocity/2(qj), w_H_root_link1/1(qj)
  w_H_root_link1/1(w_H_root) -> xCom1/2(w_H_b), stateMachineFCN/10(r_sole_H_b)
  w_H_root_link4/1(w_H_root) -> COM linear velocity/1(w_H_b), Forward Kinematics1/1, Forward Kinematics/1, Step Recovery reference generator/5(w_H_base), stateMachineFCN/9(l_sole_H_b), xCom/2(w_H_b)
  nu/1(vb + Dqj) -> vb + Dqj/1, Memory/1
  xCom1/1(xCom) -> stateMachineFCN/6(r_sole_CoM)
  stateMachineFCN/1(w_H_b) -> Visualize hom transf5/2(H), nu/2(w_H_b), w_H_b/1
  left_foot_wrench/1 -> "Visualise external wrenches  "/1(wL_WBDT), stateMachineFCN/2(wrench_leftFoot)  "wL_WBDT"
  stateMachineFCN/4(constraints) -> LEFT_RIGHT_FOOT_IN_CONTACT/1, Step Recovery reference generator/7(Constraints), nu/3("constraints ")  "constraintsSmooth"
  stateMachineFCN/8(currentState) -> state/1, Step Recovery reference generator/8(STATE), Visualize hom transf5/1("State ")
  Constant1/1 -> Mux2/2
  Mux2/1 -> CoMrefs/1
  stateMachineFCN/2(CoMDes) -> Add to bus/1(In1), Mux2/1
  stateMachineFCN/3(qDes) -> qDes/1
  Clock1/1 -> stateMachineFCN/8(t)
  holder 2/1 -> stateMachineFCN/4(q0)
  holder 1/1 -> stateMachineFCN/3(CoM_0)
  xCom/1(xCom) -> Step Recovery reference generator/1(COMx), stateMachineFCN/5(l_sole_CoM), holder 1/1
  right_foot_wrench/1 -> "Visualise external wrenches  "/2(wR_WBDT), stateMachineFCN/1(wrench_rightFoot)  "wR_WBDT"
  Switch/1(Out1) -> stateMachineFCN/11(STEP_DOWN)
  COM linear velocity/1(COM lin vel) -> Scope/1, Step Recovery reference generator/2(CoM lin vel), stateMachineFCN/12(COM_l_v)
  stateMachineFCN/10(QP_OFF) -> QP_OFF/1
  stateMachineFCN/11(SMOOTH) -> SMOOTH/1
  Memory/1 -> COM linear velocity/3(nu), Step Recovery reference generator/4(nu)
  stateMachineFCN/12(SMOOTH_com) -> SMOOTH_com/1
  Selector1/1 -> stateMachineFCN/16(COM_ref)
  chest_wrench/1 -> "Visualise external wrenches  "/3(CHEST_WBDT)
  "q_smoothed "/1 -> Step Recovery reference generator/3("q_smoothed ")
  Step Recovery reference generator/1(r_CMP) -> stateMachineFCN/13(r_CxP)
  Step Recovery reference generator/2(STEP) -> Safety Switch/1(STEP)
  Step Recovery reference generator/3(q_ref) -> stateMachineFCN/15(q_step)
  Step Recovery reference generator/4(COM_step_ref) -> Selector1/1
  Forward Kinematics1/1 -> Selector2/1, Step Recovery reference generator/10(w_H_rsole)
  Forward Kinematics/1 -> Selector/1, Step Recovery reference generator/9(w_H_lsole)
  Selector/1 -> stateMachineFCN/17(l_solex)
  Selector2/1 -> stateMachineFCN/18(r_solex)
  Step Recovery reference generator/5(CoP_ref) -> CoP_ref/1
  Step Recovery reference generator/6(MPC_ref) -> Add to bus/2(In2)
  Add to bus/1(Out1) -> MPC_ref/1
  Safety Switch/1(MAKE_A_STEP) -> stateMachineFCN/14(MAKE_A_STEP)
  Sum/1 -> stateMachineFCN/19(MPC_DECIDE_STEP)
  Constant/1 -> Product/1
  MPC_STEP/1 -> Sum/2
  Product/1 -> Sum/1
  Constant2/1 -> Product/2

== system stepRecovery/Dump and visualize/ZMPs ==
  fDesQP : Inport
  Demux1 : Demux  Outputs=3
  Demux2 : Demux  Outputs=3
  Divide{4..7} (4 alike) : Product  Inputs=*/
  Gain3 : Gain  Gain=-1
  Gain4 : Gain  Gain=-1
  Mux : Mux  Inputs=2
  Mux1 : Mux  Inputs=2
  fz taux tauy Left : Selector  InputPortWidth=12  IndexOptions=Index vector (dialog)  Indices=[3 4 5]  OutputSizes=1
  fz taux tauy Right : Selector  InputPortWidth=12  IndexOptions=Index vector (dialog)  Indices=[9 10 11]  OutputSizes=1
  ZMP_LeftFoot : Outport
  ZMP_RightFoot : Outport  Port=2
  wires:
  fz taux tauy Left/1 -> Demux1/1
  Demux1/1 -> Divide4/2, Divide5/2
  Divide7/1 -> Gain4/1
  Divide4/1 -> Mux/2
  Divide5/1 -> Gain3/1
  fz taux tauy Right/1 -> Demux2/1
  Demux2/1 -> Divide6/2, Divide7/2
  fDesQP/1 -> fz taux tauy Left/1, fz taux tauy Right/1
  Gain3/1 -> Mux/1
  Mux/1 -> ZMP_LeftFoot/1
  Divide6/1 -> Mux1/2
  Gain4/1 -> Mux1/1
  Mux1/1 -> ZMP_RightFoot/1
  Demux1/2 -> Divide4/1  "tauxL"
  Demux1/3 -> Divide5/1  "tauyL"
  Demux2/2 -> Divide6/1  "tauxR"
  Demux2/3 -> Divide7/1  "tauyR"

== system stepRecovery/Dump and visualize/plotNorms ==
  qTile_LeftLeg : Inport
  qTile_RightLeg : Inport  Port=2
  state : Inport  Port=3
  Constant : Constant  Value=sm.joints.thresholdInContact
  Constant2 : Constant  Value=sm.joints.thresholdNotInContact
  Mux : Mux  Inputs=3
  Mux1 : Mux  Inputs=3
  norm : MATLAB Function  TreatAsAtomicUnit=on
  norm(qTilde) : Scope  NumInputPorts=3
  norm1 : MATLAB Function  TreatAsAtomicUnit=on
  wires:
  Constant/1 -> Mux1/2, Mux/2  "thresholdInContact"
  qTile_LeftLeg/1 -> norm1/1(u)
  qTile_RightLeg/1 -> norm/1(u)
  norm/1(normU) -> Mux1/1  "norm(qTilde_RightL)"
  norm1/1(normU) -> Mux/1  "norm(qTilde_LeftL)"
  Mux/1 -> norm(qTilde)/1
  Mux1/1 -> norm(qTilde)/2
  Constant2/1 -> Mux1/3, Mux/3  "thresholdNotInContact"
  state/1 -> norm(qTilde)/3

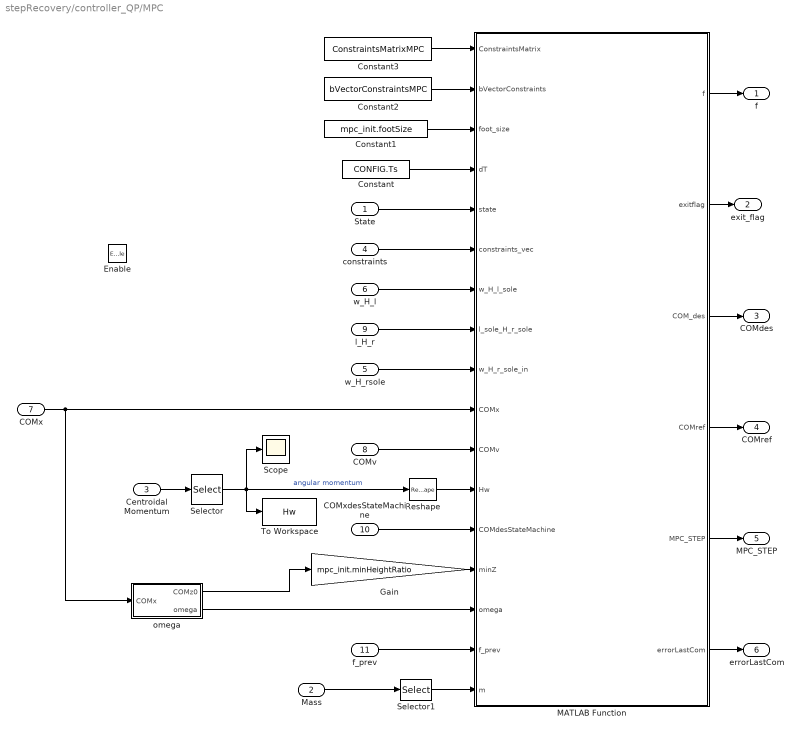
== system stepRecovery/controller_QP/MPC  ==
  State : Inport
  Mass : Inport  Port=2
  Centroidal Momentum : Inport  Port=3
  "constraints " : Inport  Port=4
  w_H_rsole : Inport  Port=5
  w_H_l : Inport  Port=6
  "COMx " : Inport  Port=7
  COMv : Inport  Port=8
  l_H_r : Inport  Port=9
  COMxdesStateMachine : Inport  Port=10
  f_prev : Inport  Port=11
  Enable : EnablePort
  Constant : Constant  Value=CONFIG.Ts
  Constant1 : Constant  Value=mpc_init.footSize
  Constant2 : Constant  Value=bVectorConstraintsMPC
  Constant3 : Constant  Value=ConstraintsMatrixMPC
  Gain : Gain  Gain=mpc_init.minHeightRatio
  MATLAB Function : MATLAB Function  TreatAsAtomicUnit=on
  Reshape : Reshape  OutputDimensionality=Column vector (2-D)
  Scope : Scope
  Selector : Selector  InputPortWidth=6  IndexOptions=Index vector (dialog)  Indices=[4:6]  OutputSizes=1
  Selector1 : Selector  NumberOfDimensions=2  InputPortWidth=3  IndexOptions=Index vector (dialog),Index vector (dialog)  Indices=1,1  OutputSizes=1,1
  To Workspace : ToWorkspace  VariableName=Hw  SampleTime=-1
      settings: Save2DSignal=2-D array (concatenate along first dimension)
  omega : Subsystem
  f : Outport
  "exit_flag " : Outport  Port=2
  COMdes : Outport  Port=3
  COMref : Outport  Port=4
  MPC_STEP : Outport  Port=5
  errorLastCom : Outport  Port=6
  wires:
  Centroidal Momentum/1 -> Selector/1
  Selector/1 -> To Workspace/1, Scope/1, Reshape/1  "angular momentum"
  "COMx "/1 -> omega/1(COMx), MATLAB Function/10(COMx)
  "constraints "/1 -> MATLAB Function/6(constraints_vec)
  w_H_l/1 -> MATLAB Function/7(w_H_l_sole)
  State/1 -> MATLAB Function/5(state)
  Selector1/1 -> MATLAB Function/17(m)
  Mass/1 -> Selector1/1
  omega/2(omega) -> MATLAB Function/15(omega)
  COMxdesStateMachine/1 -> MATLAB Function/13(COMdesStateMachine)
  COMv/1 -> MATLAB Function/11(COMv)
  w_H_rsole/1 -> MATLAB Function/9(w_H_r_sole_in)
  l_H_r/1 -> MATLAB Function/8(l_sole_H_r_sole)
  f_prev/1 -> MATLAB Function/16(f_prev)
  MATLAB Function/1(f) -> f/1
  MATLAB Function/2(exitflag) -> "exit_flag "/1
  MATLAB Function/3(COM_des) -> COMdes/1
  Constant/1 -> MATLAB Function/4(dT)
  Constant1/1 -> MATLAB Function/3(foot_size)
  Constant2/1 -> MATLAB Function/2(bVectorConstraints)
  Constant3/1 -> MATLAB Function/1(ConstraintsMatrix)
  MATLAB Function/4(COMref) -> COMref/1
  Gain/1 -> MATLAB Function/14(minZ)
  omega/1(COMz0) -> Gain/1
  Reshape/1 -> MATLAB Function/12(Hw)
  MATLAB Function/5(MPC_STEP) -> MPC_STEP/1
  MATLAB Function/6(errorLastCom) -> errorLastCom/1

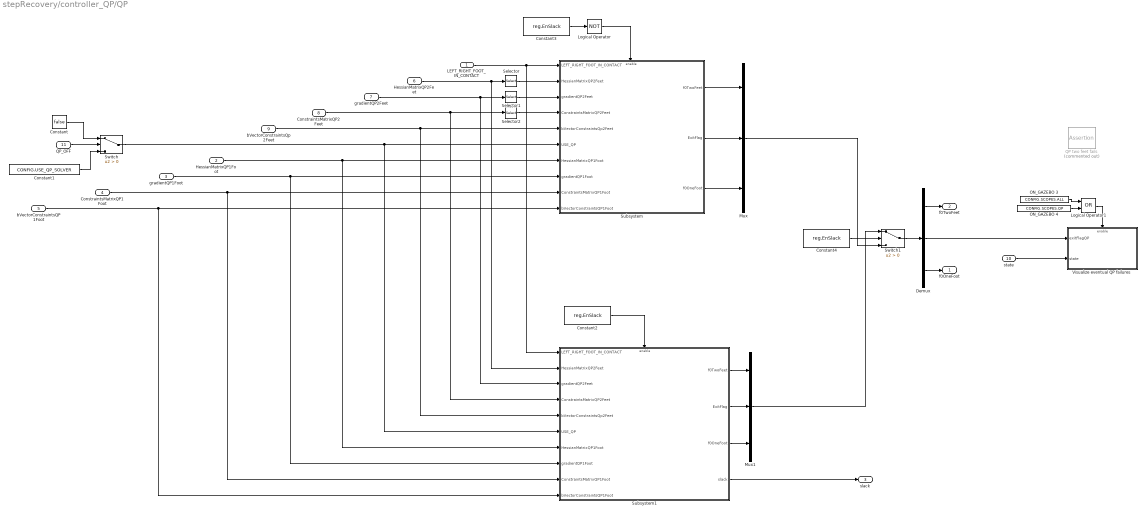
== system stepRecovery/controller_QP/QP ==
  LEFT_RIGHT_FOOT_IN_CONTACT : Inport
  HessianMatrixQP1Foot : Inport  Port=2
  gradientQP1Foot : Inport  Port=3
  ConstraintsMatrixQP1Foot : Inport  Port=4
  bVectorConstraintsQP1Foot : Inport  Port=5
  HessianMatrixQP2Feet : Inport  Port=6
  gradientQP2Feet : Inport  Port=7
  ConstraintsMatrixQP2Feet : Inport  Port=8
  bVectorConstraintsQp2Feet : Inport  Port=9
  state : Inport  Port=10
  QP_OFF : Inport  Port=11
  Constant : Constant  Value=false
  Constant1 : Constant  Value=CONFIG.USE_QP_SOLVER
  Constant2 : Constant  Value=reg.EnSlack
  Constant3 : Constant  Value=reg.EnSlack
  Constant4 : Constant  Value=reg.EnSlack
  Demux : Demux  Outputs=[12,1,12]
  Logical Operator : Logic  Operator=NOT  AllPortsSameDT=off  OutDataTypeStr=boolean
  Logical Operator1 : Logic  Operator=OR  AllPortsSameDT=off  OutDataTypeStr=boolean
  Mux : Mux  Inputs=3
  Mux1 : Mux  Inputs=3
  ON_GAZEBO 3 : Constant  Value=CONFIG.SCOPES.ALL
  ON_GAZEBO 4 : Constant  Value=CONFIG.SCOPES.QP
  QP two feet fails : Assertion  Commented=on
  Selector : Selector  NumberOfDimensions=2  InputPortWidth=3  IndexOptions=Index vector (dialog),Index vector (dialog)  Indices=[1:12],[1:12]  OutputSizes=1,1
  Selector1 : Selector  InputPortWidth=18  IndexOptions=Index vector (dialog)  Indices=[1:12]  OutputSizes=1
  Selector2 : Selector  NumberOfDimensions=2  InputPortWidth=18  IndexOptions=Index vector (dialog),Index vector (dialog)  Indices=[1:38],[1:12]  OutputSizes=1,1
  Subsystem : Subsystem
  Subsystem1 : Subsystem
  Switch : Switch  Criteria=u2 > Threshold
  Switch1 : Switch  Criteria=u2 > Threshold
  Visualize eventual QP failures : Subsystem
  f0OneFoot : Outport
  f0TwoFeet : Outport  Port=2
  slack : Outport  Port=3
  wires:
  Logical Operator1/1 -> Visualize eventual QP failures/Enable
  state/1 -> Visualize eventual QP failures/2(state)
  Constant1/1 -> Switch/3
  ON_GAZEBO 3/1 -> Logical Operator1/1
  ON_GAZEBO 4/1 -> Logical Operator1/2
  QP_OFF/1 -> Switch/2
  Constant/1 -> Switch/1
  Subsystem1/4(slack) -> slack/1
  LEFT_RIGHT_FOOT_IN_CONTACT/1 -> Subsystem1/1(LEFT_RIGHT_FOOT_IN_CONTACT), Subsystem/1(LEFT_RIGHT_FOOT_IN_CONTACT)
  HessianMatrixQP2Feet/1 -> Subsystem1/2(HessianMatrixQP2Feet), Selector/1
  gradientQP2Feet/1 -> Subsystem1/3(gradientQP2Feet), Selector1/1
  ConstraintsMatrixQP2Feet/1 -> Subsystem1/4(ConstraintsMatrixQP2Feet), Selector2/1
  bVectorConstraintsQp2Feet/1 -> Subsystem1/5(bVectorConstraintsQp2Feet), Subsystem/5(bVectorConstraintsQp2Feet)
  Switch/1 -> Subsystem1/6(USE_QP), Subsystem/6(USE_QP)
  HessianMatrixQP1Foot/1 -> Subsystem1/7(HessianMatrixQP1Foot), Subsystem/7(HessianMatrixQP1Foot)
  gradientQP1Foot/1 -> Subsystem1/8(gradientQP1Foot), Subsystem/8(gradientQP1Foot)
  ConstraintsMatrixQP1Foot/1 -> Subsystem1/9(ConstraintsMatrixQP1Foot), Subsystem/9(ConstraintsMatrixQP1Foot)
  bVectorConstraintsQP1Foot/1 -> Subsystem1/10(bVectorConstraintsQP1Foot), Subsystem/10(bVectorConstraintsQP1Foot)
  Constant2/1 -> Subsystem1/Enable
  Constant3/1 -> Logical Operator/1
  Logical Operator/1 -> Subsystem/Enable
  Subsystem/1(f0TwoFeet) -> Mux/1
  Subsystem/2(ExitFlag) -> Mux/2
  Subsystem/3(f0OneFoot) -> Mux/3
  Subsystem1/2(ExitFlag) -> Mux1/2
  Subsystem1/1(f0TwoFeet) -> Mux1/1
  Subsystem1/3(f0OneFoot) -> Mux1/3
  Constant4/1 -> Switch1/2
  Mux1/1 -> Switch1/1
  Mux/1 -> Switch1/3
  Switch1/1 -> Demux/1
  Demux/1 -> f0TwoFeet/1
  Demux/3 -> f0OneFoot/1
  Demux/2 -> Visualize eventual QP failures/1(exitFlagQP)
  Selector/1 -> Subsystem/2(HessianMatrixQP2Feet)
  Selector1/1 -> Subsystem/3(gradientQP2Feet)
  Selector2/1 -> Subsystem/4(ConstraintsMatrixQP2Feet)

== system stepRecovery/controller_QP/integralOf Hw ==
  qjDes : Inport
  qj : Inport  Port=2
  Centroidal Momentum : WBToolboxLibrary/wholeBodyModel/Dynamics/Centroidal Momentum  robotName=WBT_robotName  localName=WBT_modelName  wbiFile=WBT_wbiFilename  wbiList=WBT_wbiList
  Jacobian : WBToolboxLibrary/wholeBodyModel/Jacobians/Jacobian  frameName='l_sole'  robotName=WBT_robotName  localName=WBT_modelName  wbiFile=WBT_wbiFilename  wbiList=WBT_wbiList
  MATLAB Function : MATLAB Function  TreatAsAtomicUnit=on
  MATLAB Function1 : MATLAB Function  TreatAsAtomicUnit=on
  Sum : Sum  Inputs=|-+
  l_sole_H_root_link : Subsystem
  intHw : Outport
  wires:
  qjDes/1 -> l_sole_H_root_link/1(qj0), Centroidal Momentum/2, Jacobian/2, Sum/1
  l_sole_H_root_link/1(l_sole_H_root_link) -> Centroidal Momentum/1, Jacobian/1
  qj/1 -> Sum/2
  Sum/1 -> MATLAB Function/1(qjErr)
  MATLAB Function/1(dqjEquivalent) -> Centroidal Momentum/4
  MATLAB Function/2(vbEquivalent) -> Centroidal Momentum/3
  Jacobian/1 -> MATLAB Function/2(Jc)
  Centroidal Momentum/1 -> MATLAB Function1/1(H)
  MATLAB Function1/1(deltaPhi) -> intHw/1

== system stepRecovery/controller_QP/xCom ==
  w_H_b : Inport
  qj : Inport  Port=2
  "CoM6D ->  CoMXYZ2" : Selector  NumberOfDimensions=2  InputPortWidth=7  IndexOptions=Index vector (dialog),Index vector (dialog)  Indices=[1 2 3],[4]  OutputSizes=1,1
  com : WBToolboxLibrary/wholeBodyModel/Kinematics/Forward Kinematics  frameName='com'  robotName=WBT_robotName  localName=WBT_modelName  wbiFile=WBT_wbiFilename  wbiList=WBT_wbiList
  xCom : Outport
  wires:
  qj/1 -> com/2
  "CoM6D ->  CoMXYZ2"/1 -> xCom/1
  com/1 -> "CoM6D ->  CoMXYZ2"/1
  w_H_b/1 -> com/1

== system stepRecovery/synchronizer/GAZEBO_SYNCHRONIZER ==
  Enable : EnablePort
  Simulator Synchronizer : WBToolboxLibrary/Utilities/Simulator Synchronizer  period=CONFIG.Ts  serverPortName='/clock/rpc'  clientPortName='/WBT_synchronizer/rpc:o'

== system stepRecovery/synchronizer/REAL_TIME_SYNC ==
  Enable : EnablePort
  Real Time Synchronizer : WBToolboxLibrary/Utilities/Real Time Synchronizer  period=CONFIG.Ts

== system stepRecovery/DesValues/State Machine Step Recovery/Add to bus ==
  In1 : Inport
  In2 : Inport  Port=2
  Bus Creator : BusCreator  Inputs=4
  Bus Selector : BusSelector  OutputSignals=Step,l_sole_H_r_sole,Enable
  Out1 : Outport
  wires:
  In2/1 -> Bus Selector/1
  Bus Selector/1 -> Bus Creator/2  "<Step>"
  In1/1 -> Bus Creator/1  "COMxdes"
  Bus Selector/2 -> Bus Creator/3  "<l_sole_H_r_sole>"
  Bus Selector/3 -> Bus Creator/4  "<Enable>"
  Bus Creator/1 -> Out1/1

== system stepRecovery/DesValues/State Machine Step Recovery/COM linear velocity ==
  w_H_b : Inport
  qj : Inport  Port=2
  nu : Inport  Port=3
  Jacobian : WBToolboxLibrary/wholeBodyModel/Jacobians/Jacobian  frameName='com'  robotName=WBT_robotName  localName=WBT_modelName  wbiFile=WBT_wbiFilename  wbiList=WBT_wbiList
  Matrix Multiply : Product  Multiplication=Matrix(*)
  Selector1 : Selector  InputPortWidth=6  IndexOptions=Index vector (dialog)  Indices=[1:3]  OutputSizes=1
  COM lin vel : Outport
  wires:
  qj/1 -> Jacobian/2
  w_H_b/1 -> Jacobian/1
  Selector1/1 -> COM lin vel/1
  Jacobian/1 -> Matrix Multiply/1
  nu/1 -> Matrix Multiply/2
  Matrix Multiply/1 -> Selector1/1

== system stepRecovery/DesValues/State Machine Step Recovery/Safety Switch ==
  STEP : Inport
  Constant : Constant  Value=0
  Manual Switch : ManualSwitch  CurrentSetting=0
  MAKE_A_STEP : Outport
  wires:
  STEP/1 -> Manual Switch/2
  Manual Switch/1 -> MAKE_A_STEP/1
  Constant/1 -> Manual Switch/1
